simulink model "Sim_Helikopter"  (R2020b)
settings: Solver=ode113  StartTime=0.0  StopTime=50  RelTol=1e-2  EnableMultiTasking=on
PostLoadFcn:
  | , if any(exist('dsrtsu_mdlpostloadfcn', 'file') == [2, 3, 6]), try dsrtsu_mdlpostloadfcn('Execute', bdroot); catch fprintf('Error in PostLoadFcn (dsrtsu_mdlpostloadfcn) for model "%s":\n %s\n', bdroot, lasterr); end, end,
values from neighbouring files (symbols this model uses):
  initCond = [0,0,q20,0,0,0,0,0,0,0,0,0]'    [set_parameter_vollstaendigesModell.m]
undefined symbols (not defined in the file or in its folder): regPar, sysPar, Ta
libraries: simulink x1
settings Model: DSRTSU_INTERNAL_RTI_VER=480  DSRTSU_INTERNAL_RTI_TYPE=rti1202  DSRTSU_INTERNAL_RTIFPGA=70  ExtModeArmWhenConnect=off  Creator=tk  LastModifiedBy=paul
settings DataIOCC: LimitDataPoints=on  SaveFormat=Array  SignalLoggingSaveFormat=ModelDataLogs  ReturnWorkspaceOutputs=off  SignalLoggingName=sigsOut
settings OptimizationCC: ConditionallyExecuteInputs=off  OptimizeBlockIOStorage=off  BufferReuse=off  GlobalBufferReuse=off  ExpressionFolding=off  ExpressionDepthLimit=2147483647  LocalBlockOutputs=off  InitFltsAndDblsToZero=on  LifeSpan=inf  OptimizeDataStoreBuffers=off  BusAssignmentInplaceUpdate=off
settings DebuggingCC: SaveWithParameterizedLinksMsg=none  UnderspecifiedInitializationDetection=Classic  MergeDetectMultiDrivingBlocksExec=none  SignalResolutionControl=TryResolveAllWithWarning  MultiTaskDSMMsg=warning  MultiTaskCondExecSysMsg=none  FcnCallInpInsideContextMsg=warning  AllowSymbolicDim=off  StateNameClashWarn=warning  SFUnexpectedBacktrackingDiag=warning  SFNoUnconditionalDefaultTransitionDiag=warning  SFExecutionAtInitializationDiag=none  ArithmeticOperatorsInVariantConditions=warning
settings HardwareCC: ProdBitPerPointer=32  ProdBitPerSizeT=32  ProdBitPerPtrDiffT=32  ProdLargestAtomicFloat=None  ProdIntDivRoundTo=Undefined  ProdEndianess=Unspecified  ProdWordSize=32  ProdHWDeviceType=32-bit Generic  TargetBitPerLong=64  TargetBitPerPointer=64  TargetBitPerSizeT=64  TargetBitPerPtrDiffT=64  TargetLongLongMode=on  TargetIntDivRoundTo=Zero  TargetEndianess=LittleEndian  TargetWordSize=64  TargetHWDeviceType=MATLAB Host  ProdEqTarget=off
settings ModelReferenceCC: PropagateSignalLabelsOutOfModel=off
settings SFSimCC: SimUseLocalCustomCode=off  SimParseCustomCode=off  CustomCodeUndefinedFunction=UseInterfaceOnly
settings RTWCC: Description=S-function Target  SystemTargetFile=rtwsfcn.tlc  TemplateMakefile=rtwsfcn_default_tmf  RetainRTWFile=on  RTWUseLocalCustomCode=off  RTWCompilerOptimization=on
settings CodeAppCC: StateflowObjectComments=on
settings STFCustomTargetCC: ModelReferenceCompliant=off  CompOptLevelCompliant=on  ConcurrentExecutionCompliant=off  MATLABClassNameForMDSCustomization=Simulink.SoftwareTarget.TargetSpecificTriggerConfigurationBase  CPPClassGenCompliant=off  SystemTargetFile=rtwsfcn.tlc
settings ConfigComp: CovMetricSettings=dw  CovSaveCumulativeToWorkspaceVar=on  CovSaveSingleToWorkspaceVar=on  CovExternalEMLEnable=off

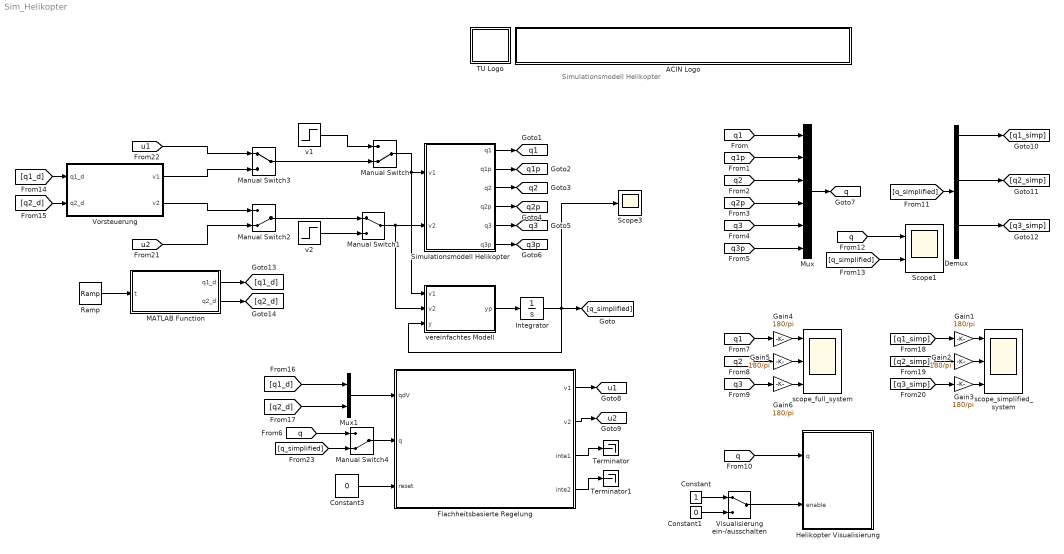
== system Sim_Helikopter ==
  note: Simulationsmodell Helikopter
  ACIN Logo : Subsystem
      mask init:
      | s = get_param(gcb,'UserData');
      mask Display:
      | image(s.logo,[0 0 439 45]);
      | %axis image
  Constant : Constant
  Constant1 : Constant  Value=0
  Constant3 : Constant  Value=0
  Demux : Demux  Outputs=6
  Flachheitsbasierte Regelung : MATLAB Function  TreatAsAtomicUnit=on
  Gain{1..6} (6 alike) : Gain  Gain=180/pi  SaturateOnIntegerOverflow=on  OutDataTypeStr=Inherit: Same as input  ParamDataTypeStr=Inherit: Same as input
  Helikopter Visualisierung : MATLAB Function  TreatAsAtomicUnit=on
  Integrator : Integrator  InitialCondition=sysPar.qR
  MATLAB Function : MATLAB Function  TreatAsAtomicUnit=on
  Manual Switch : ManualSwitch  CurrentSetting=0
  Manual Switch1 : ManualSwitch
  Manual Switch2 : ManualSwitch  CurrentSetting=0
  Manual Switch3 : ManualSwitch
  Manual Switch4 : ManualSwitch  CurrentSetting=0
  Mux : Mux  Inputs=6
  Mux1 : Mux  Inputs=2
  Ramp : simulink/Sources/Ramp  slope=1  start=0  InitialOutput=0
  Scope1 : Scope  NumInputPorts=2
  Scope3 : Scope
  Simulationsmodell Helikopter : Subsystem
      settings: MinAlgLoopOccurrences=on
  TU Logo : Subsystem
      mask init:
      | s = get_param(gcb,'UserData');
      mask Display: image(s.logo,[0 0 45 45]);
  Terminator : Terminator
  Terminator1 : Terminator
  Visualisierung ein-/ausschalten : ManualSwitch
  Vorsteuerung : MATLAB Function  TreatAsAtomicUnit=on
  scope_full_system : Scope  NumInputPorts=3
  scope_simplified_system : Scope  NumInputPorts=3
  v1 : Step  After=.5  SampleTime=0
  v2 : Step  After=0  SampleTime=0
  vereinfachtes Modell : MATLAB Function  TreatAsAtomicUnit=on
  tag scope: q1=global, q1p=global, q2=global, q2p=global, q3=global, q3p=global, q=global, u1=global, u2=global
  wires:
  Gain4/1 -> scope_full_system/1
  Gain5/1 -> scope_full_system/2
  Gain6/1 -> scope_full_system/3
  Flachheitsbasierte Regelung/1(v1) -> [u1]
  Flachheitsbasierte Regelung/2(v2) -> [u2]
  Constant3/1 -> Flachheitsbasierte Regelung/3(reset)
  Simulationsmodell Helikopter/1(q1) -> [q1]
  Simulationsmodell Helikopter/2(q1p) -> [q1p]
  Simulationsmodell Helikopter/3(q2) -> [q2]
  Simulationsmodell Helikopter/4(q2p) -> [q2p]
  Simulationsmodell Helikopter/5(q3) -> [q3]
  Simulationsmodell Helikopter/6(q3p) -> [q3p]
  Mux/1 -> [q]
  [q1] -> Mux/1
  [q1p] -> Mux/2
  [q2] -> Mux/3
  [q2p] -> Mux/4
  [q3] -> Mux/5
  [q3p] -> Mux/6
  [q1] -> Gain4/1
  [q2] -> Gain5/1
  [q3] -> Gain6/1
  Flachheitsbasierte Regelung/3(inte1) -> Terminator/1
  Flachheitsbasierte Regelung/4(inte2) -> Terminator1/1
  Visualisierung ein-/ausschalten/1 -> Helikopter Visualisierung/2(enable)
  Constant/1 -> Visualisierung ein-/ausschalten/1
  [q] -> Helikopter Visualisierung/1(q)
  Constant1/1 -> Visualisierung ein-/ausschalten/2
  vereinfachtes Modell/1(yp) -> Integrator/1
  Integrator/1 -> Scope3/1, [q_simplified], vereinfachtes Modell/3(y)
  [q_simplified] -> Demux/1
  Demux/1 -> [q1_simp]
  Demux/3 -> [q2_simp]
  Demux/5 -> [q3_simp]
  [q] -> Scope1/1
  [q_simplified] -> Scope1/2
  Ramp/1 -> MATLAB Function/1(t)
  MATLAB Function/1(q1_d) -> [q1_d]
  MATLAB Function/2(q2_d) -> [q2_d]
  [q1_d] -> Vorsteuerung/1(q1_d)
  [q2_d] -> Vorsteuerung/2(q2_d)
  Manual Switch/1 -> vereinfachtes Modell/1(v1), Simulationsmodell Helikopter/1(v1)
  v1/1 -> Manual Switch/1
  Manual Switch1/1 -> vereinfachtes Modell/2(v2), Simulationsmodell Helikopter/2(v2)
  v2/1 -> Manual Switch1/2
  Mux1/1 -> Flachheitsbasierte Regelung/1(qdV)
  [q1_d] -> Mux1/1
  [q2_d] -> Mux1/2
  Gain3/1 -> scope_simplified_system/3
  [q3_simp] -> Gain3/1
  Gain2/1 -> scope_simplified_system/2
  Gain1/1 -> scope_simplified_system/1
  [q1_simp] -> Gain1/1
  [q2_simp] -> Gain2/1
  Manual Switch2/1 -> Manual Switch1/1
  Manual Switch3/1 -> Manual Switch/2
  [u1] -> Manual Switch3/1
  Vorsteuerung/1(v1) -> Manual Switch3/2
  [u2] -> Manual Switch2/2
  Vorsteuerung/2(v2) -> Manual Switch2/1
  [q_simplified] -> Manual Switch4/2
  Manual Switch4/1 -> Flachheitsbasierte Regelung/2(q)
  [q] -> Manual Switch4/1

== system Sim_Helikopter/ACIN Logo ==

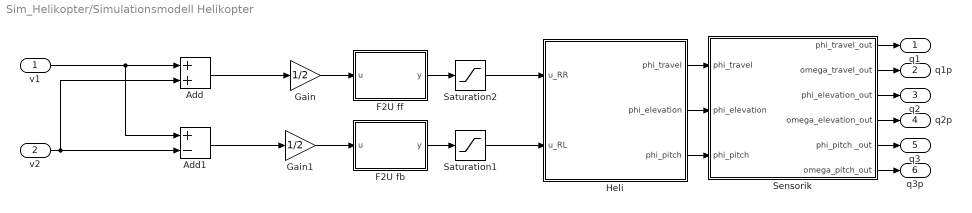
== system Sim_Helikopter/Simulationsmodell Helikopter ==
  v1 : Inport
  v2 : Inport  Port=2
  Add : Sum
  Add1 : Sum  Inputs=+-
  F2U fb : MATLAB Function  TreatAsAtomicUnit=on
  F2U ff : MATLAB Function  TreatAsAtomicUnit=on
  Gain : Gain  Gain=1/2
  Gain1 : Gain  Gain=1/2
  Heli : Subsystem
  Saturation1 : Saturate  UpperLimit=15  LowerLimit=-15
  Saturation2 : Saturate  UpperLimit=15  LowerLimit=-15
  Sensorik : Subsystem
  q1 : Outport  VectorParamsAs1DForOutWhenUnconnected=off
  q1p : Outport  Port=2  VectorParamsAs1DForOutWhenUnconnected=off
  q2 : Outport  Port=3  VectorParamsAs1DForOutWhenUnconnected=off
  q2p : Outport  Port=4  VectorParamsAs1DForOutWhenUnconnected=off
  q3 : Outport  Port=5  VectorParamsAs1DForOutWhenUnconnected=off
  q3p : Outport  Port=6  VectorParamsAs1DForOutWhenUnconnected=off
  wires:
  Saturation1/1 -> Heli/2(u_RL)
  Saturation2/1 -> Heli/1(u_RR)
  Heli/1(phi_travel) -> Sensorik/1(phi_travel)
  Heli/2(phi_elevation) -> Sensorik/2(phi_elevation)
  Heli/3(phi_pitch) -> Sensorik/3(phi_pitch)
  Sensorik/1(phi_travel_out) -> q1/1
  Sensorik/2(omega_travel_out) -> q1p/1
  Sensorik/3(phi_elevation_out) -> q2/1
  Sensorik/4(omega_elevation_out) -> q2p/1
  Sensorik/5(phi_pitch _out) -> q3/1
  Sensorik/6(omega_pitch_out) -> q3p/1
  v1/1 -> Add/1, Add1/1
  v2/1 -> Add/2, Add1/2
  Add/1 -> Gain/1
  Add1/1 -> Gain1/1
  Gain/1 -> F2U ff/1(u)
  Gain1/1 -> F2U fb/1(u)
  F2U ff/1(y) -> Saturation2/1
  F2U fb/1(y) -> Saturation1/1

== system Sim_Helikopter/TU Logo ==

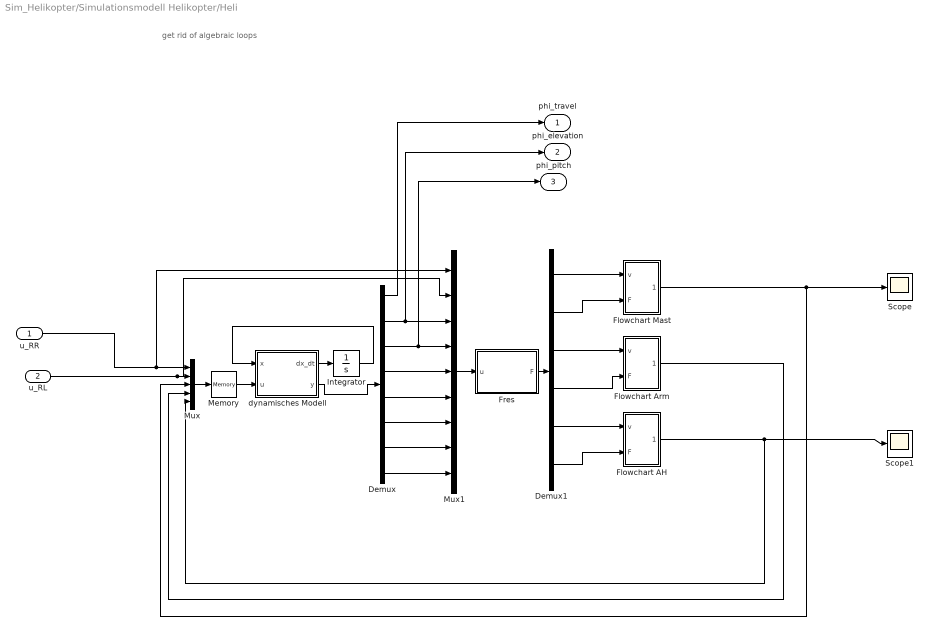
== system Sim_Helikopter/Simulationsmodell Helikopter/Heli ==
  note: get rid of algebraic loops
  u_RR : Inport
  u_RL : Inport  Port=2
  Demux : Demux  Outputs=8
      settings: DisplayOption=none
  Demux1 : Demux  Outputs=6
      settings: DisplayOption=none
  Flowchart AH : Subsystem
  Flowchart Arm : Subsystem
  Flowchart Mast : Subsystem
  Fres : MATLAB Function  TreatAsAtomicUnit=on
  Integrator : Integrator  InitialCondition=initCond
  Memory : Memory
  Mux : Mux  Inputs=5
  Mux1 : Mux  Inputs=9
  Scope : Scope
  Scope1 : Scope
  dynamisches Modell : MATLAB Function  TreatAsAtomicUnit=on
  phi_travel : Outport  VectorParamsAs1DForOutWhenUnconnected=off
  phi_elevation : Outport  Port=2  VectorParamsAs1DForOutWhenUnconnected=off
  phi_pitch : Outport  Port=3  VectorParamsAs1DForOutWhenUnconnected=off
  wires:
  Demux/1 -> phi_travel/1
  u_RR/1 -> Mux1/1, Mux/1
  u_RL/1 -> Mux1/2, Mux/2
  Demux1/6 -> Flowchart AH/2(F)
  Demux1/5 -> Flowchart AH/1(v)
  Demux1/4 -> Flowchart Arm/2(F)
  Demux1/3 -> Flowchart Arm/1(v)
  Demux1/2 -> Flowchart Mast/2(F)
  Demux1/1 -> Flowchart Mast/1(v)
  Fres/1(F) -> Demux1/1
  Mux1/1 -> Fres/1(u)
  Demux/2 -> Mux1/3, phi_elevation/1
  Demux/3 -> Mux1/4, phi_pitch/1
  Demux/4 -> Mux1/5
  Demux/5 -> Mux1/6
  Demux/6 -> Mux1/7
  Demux/7 -> Mux1/8
  Demux/8 -> Mux1/9
  dynamisches Modell/2(y) -> Demux/1
  Mux/1 -> Memory/1
  dynamisches Modell/1(dx_dt) -> Integrator/1
  Integrator/1 -> dynamisches Modell/1(x)
  Flowchart AH/1(Out1) -> Scope1/1, Mux/5
  Flowchart Arm/1(Out1) -> Mux/4
  Flowchart Mast/1(Out1) -> Mux/3, Scope/1
  Memory/1 -> dynamisches Modell/2(u)

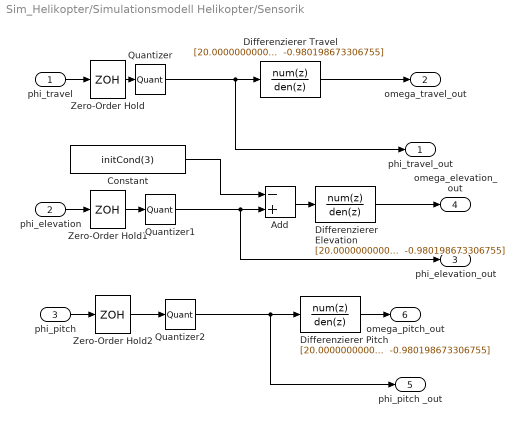
== system Sim_Helikopter/Simulationsmodell Helikopter/Sensorik ==
  phi_travel : Inport
  phi_elevation : Inport  Port=2
  phi_pitch : Inport  Port=3
  Add : Sum  Inputs=-+
  Constant : Constant  Value=initCond(3)
  Differenzierer Elevation : DiscreteTransferFcn  Numerator=[20.000000000000000 -19.999999999999996]  Denominator="[1.000000000000000  -0.980198673306755]"  SampleTime=1e-3
  Differenzierer Pitch : DiscreteTransferFcn  Numerator=[20.000000000000000 -19.999999999999996]  Denominator="[1.000000000000000  -0.980198673306755]"  SampleTime=1e-3
  Differenzierer Travel : DiscreteTransferFcn  Numerator=[20.000000000000000 -19.999999999999996]  Denominator="[1.000000000000000  -0.980198673306755]"  SampleTime=1e-3
  Quantizer : Quantizer  QuantizationInterval=2*pi/2^13
  Quantizer1 : Quantizer  QuantizationInterval=2*pi/4096
  Quantizer2 : Quantizer  QuantizationInterval=2*pi/4096
  Zero-Order Hold : ZeroOrderHold  SampleTime=1e-3
  Zero-Order Hold1 : ZeroOrderHold  SampleTime=1e-3
  Zero-Order Hold2 : ZeroOrderHold  SampleTime=1e-3
  phi_travel_out : Outport  VectorParamsAs1DForOutWhenUnconnected=off
  omega_travel_out : Outport  Port=2  VectorParamsAs1DForOutWhenUnconnected=off
  phi_elevation_out : Outport  Port=3  VectorParamsAs1DForOutWhenUnconnected=off
  omega_elevation_out : Outport  Port=4  VectorParamsAs1DForOutWhenUnconnected=off
  phi_pitch _out : Outport  Port=5  VectorParamsAs1DForOutWhenUnconnected=off
  omega_pitch_out : Outport  Port=6  VectorParamsAs1DForOutWhenUnconnected=off
  wires:
  Add/1 -> Differenzierer Elevation/1
  Constant/1 -> Add/1
  Zero-Order Hold/1 -> Quantizer/1
  Quantizer/1 -> Differenzierer Travel/1, phi_travel_out/1
  Zero-Order Hold1/1 -> Quantizer1/1
  Quantizer1/1 -> Add/2, phi_elevation_out/1
  Zero-Order Hold2/1 -> Quantizer2/1
  Quantizer2/1 -> phi_pitch _out/1, Differenzierer Pitch/1
  Differenzierer Travel/1 -> omega_travel_out/1
  phi_travel/1 -> Zero-Order Hold/1
  Differenzierer Elevation/1 -> omega_elevation_out/1
  phi_elevation/1 -> Zero-Order Hold1/1
  Differenzierer Pitch/1 -> omega_pitch_out/1
  phi_pitch/1 -> Zero-Order Hold2/1

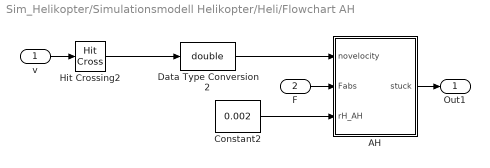
== system Sim_Helikopter/Simulationsmodell Helikopter/Heli/Flowchart AH ==
  v : Inport
  F : Inport  Port=2
  AH : Stateflow chart  TreatAsAtomicUnit=on
  Constant2 : Constant  Value=0.002
  Data Type Conversion2 : DataTypeConversion  OutDataTypeStr=double  SaturateOnIntegerOverflow=on  RndMeth=Zero
  Hit Crossing2 : HitCross  ZeroCross=off
  Out1 : Outport  VectorParamsAs1DForOutWhenUnconnected=off
  wires:
  AH/1(stuck) -> Out1/1
  F/1 -> AH/2(Fabs)
  v/1 -> Hit Crossing2/1
  Constant2/1 -> AH/3(rH_AH)
  Data Type Conversion2/1 -> AH/1(novelocity)
  Hit Crossing2/1 -> Data Type Conversion2/1

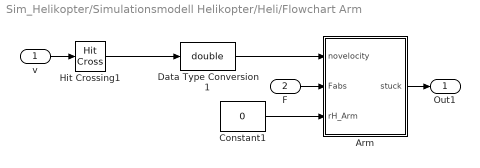
== system Sim_Helikopter/Simulationsmodell Helikopter/Heli/Flowchart Arm ==
  v : Inport
  F : Inport  Port=2
  Arm : Stateflow chart  TreatAsAtomicUnit=on
  Constant1 : Constant  Value=0
  Data Type Conversion1 : DataTypeConversion  OutDataTypeStr=double  SaturateOnIntegerOverflow=on  RndMeth=Zero
  Hit Crossing1 : HitCross  ZeroCross=off
  Out1 : Outport  VectorParamsAs1DForOutWhenUnconnected=off
  wires:
  Arm/1(stuck) -> Out1/1
  F/1 -> Arm/2(Fabs)
  v/1 -> Hit Crossing1/1
  Hit Crossing1/1 -> Data Type Conversion1/1
  Data Type Conversion1/1 -> Arm/1(novelocity)
  Constant1/1 -> Arm/3(rH_Arm)

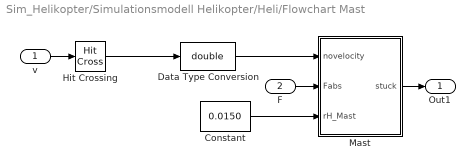
== system Sim_Helikopter/Simulationsmodell Helikopter/Heli/Flowchart Mast ==
  v : Inport
  F : Inport  Port=2
  Constant : Constant  Value=0.0150
  Data Type Conversion : DataTypeConversion  OutDataTypeStr=double  SaturateOnIntegerOverflow=on  RndMeth=Zero
  Hit Crossing : HitCross  ZeroCross=off
  Mast : Stateflow chart  TreatAsAtomicUnit=on
  Out1 : Outport  VectorParamsAs1DForOutWhenUnconnected=off
  wires:
  Mast/1(stuck) -> Out1/1
  F/1 -> Mast/2(Fabs)
  v/1 -> Hit Crossing/1
  Constant/1 -> Mast/3(rH_Mast)
  Data Type Conversion/1 -> Mast/1(novelocity)
  Hit Crossing/1 -> Data Type Conversion/1

== matlab function Sim_Helikopter/Simulationsmodell Helikopter/Heli/dynamisches Modell ==
  data: x input; u input; dx_dt output; p parameter; y output
function [dx_dt, y]= fcn(x, u, p)
%#codegen

[dx_dt, y] = heli_haft_mfun(x,u,p);

== matlab function Sim_Helikopter/Helikopter Visualisierung ==
  settings: updateMethod=DISCRETE  sampleTime=0.1
  data: q input; enable input
function visualization(q, enable)
  %Die Framerate wird durch die Sampling Time des Blocks vorgegeben.

  persistent ini; if isempty(ini);    ini = 0;    end
  persistent z12; if isempty(z12);    z12 = 1;    end
  persistent x23; if isempty(x23);    x23 = 1;    end
  persistent xh;  if isempty(xh);     xh = 1;     end
  persistent yh;  if isempty(yh);     yh = 1;     end
  persistent zh;  if isempty(zh);     zh = 1;     end
  persistent ph;  if isempty(ph);     ph = 1;     end
  
  if ~ini
    if(enable)
      h=figure(100);
      clf('reset');
      plot3(-2, -2, 0);
      plot3( 2,  2, 0);
      plot3(-2,  2, 0);
      plot3( 2, -2, 0);
      axis([-2 2 -2 2 0 1]);
      xlabel('x');
      ylabel('y');
      zlabel('-z');

      r  = 0.1;
      yn = 0.2:0.01:0.4;
      yp = 0.4:-0.01:0.2;
      a  = abs(r^2 - (yn - 0.3).^2);
      xn = -sqrt(a);
      xp =  sqrt(a);

      y2 = [yn'; yp'];
      x2 = [xn'; xp'];
      z2 = zeros(size(x2));

      yn = -0.2:-0.01:-0.4;
      yp = -0.4:0.01:-0.2;
      b  = abs(r^2 - (yn + 0.3).^2);
      xn = -sqrt(b);
      xp =  sqrt(b);

      y1 = [yn'; yp'];
      x1 = [xn'; xp'];
      z1 = zeros(size(x1));

      xh = [x1', x2'];
      yh = [y1', y2'];
      zh = [z1', z2'];
      ph = [xh; yh; zh; ones(size(zh))];
    else
      h=findobj('type','figure','Number',100);
      if(~isempty(h))
        close(h);
      end
    end
    ini = 1;
  end
  
  if(enable)
    q1=q(1);
    q2=q(3);
    q3=q(5);
    
    T02 = [-sin(q1) * cos(q2) -cos(q1) -sin(q1) * sin(q2) 0; cos(q1) * cos(q2) -sin(q1) cos(q1) * sin(q2) 0; -sin(q2) 0 cos(q2) z12; 0 0 0 1;];
    T03 = [-sin(q1) * cos(q2) cos(q1) * cos(q3) + sin(q1) * sin(q2) * sin(q3) -cos(q1) * sin(q3) + sin(q1) * sin(q2) * cos(q3) -sin(q1) * cos(q2) * x23; cos(q1) * cos(q2) sin(q1) * cos(q3) - cos(q1) * sin(q2) * sin(q3) -sin(q1) * sin(q3) - cos(q1) * sin(q2) * cos(q3) cos(q1) * cos(q2) * x23; -sin(q2) -cos(q2) * sin(q3) -cos(q2) * cos(q3) -sin(q2) * x23 + z12; 0 0 0 1;];

    clf('reset');
    % Nullzeiger
    xn = [0;1];
    yn = [0;0];
    zn = [0;0];
    plot3(xn, yn, zn);
    hold on;
    grid on;

    % Staender
    p0 = [0; 0; 0];
    p1 = [0; 0; 1];    
    lines = [p0';p1'];
    xs = lines(1:2,1);
    ys = lines(1:2,2);
    zs = lines(1:2,3);
    plot3(xs, ys, zs);

    % Balken
    p0 = T02*[1; 0; 0; 1];
    p1 = T02*[-1; 0; 0; 1];    
    lines = [p0(1:3)';p1(1:3)'];
    xb = lines(1:2,1);
    yb = lines(1:2,2);
    zb = lines(1:2,3);
    plot3(xb, yb, zb);

    % Helicopter
    lines = T03*ph;% [0; 0.2; 0; 1];
    % p1 = T03*[0; -0.2; 0; 1];    
    % lines = [p0(1:3)';p1(1:3)'];
    xh = lines(1,:);
    yh = lines(2,:);
    zh = lines(3,:);
    plot3(xh, yh, zh);

    plot3(-2, -2, 0);
    plot3( 2,  2, 0);
    plot3(-2,  2, 0);
    plot3( 2, -2, 0);
    axis([-2 2 -2 2 0 2]);

    drawnow
  end
end

== matlab function Sim_Helikopter/MATLAB Function ==
  data: t input; q1_d output; q2_d output; sysPar parameter
function [q1_d,q2_d] = Trajektorie(t,sysPar)
    
   
    beta5 = 126; beta6 = -420; beta7 = 540; beta8 = -315; beta9 = 70;
    
    % Startpunkt -> Ruhelage
    q1_0 = sysPar.qR(1);
    q2_0 = sysPar.qR(3);
    
    % Zeitpunkte und Endpunkte laut Angabe
    T1 = 5;
    T2 = 10;
    
    q1_end = 2*pi;
    q2_end = 0;

    
    q1_d = [q1_0; zeros(4,1)];
    q2_d = [q2_0; zeros(4,1)];
    
    % Ruhelage
    if (t > 0) && (t <= T1)
        q2_d(1) = q2_0 + (q2_end - q2_0) * (beta5 * t ^ 5 / T1 ^ 5 + beta6 * t ^ 6 / T1 ^ 6 + beta7 * t ^ 7 / T1 ^ 7 + beta8 * t ^ 8 / T1 ^ 8 + beta9 * t ^ 9 / T1 ^ 9);
        q2_d(5) = (q2_end - q2_0) * (120 * beta5 * t / T1 ^ 5 + 360 * beta6 * t ^ 2 / T1 ^ 6 + 840 * beta7 * t ^ 3 / T1 ^ 7 + 1680 * beta8 * t ^ 4 / T1 ^ 8 + 3024 * beta9 * t ^ 5 / T1 ^ 9);
        q2_d(4) = (q2_end - q2_0) * (60 * beta5 * t ^ 2 / T1 ^ 5 + 120 * beta6 * t ^ 3 / T1 ^ 6 + 210 * beta7 * t ^ 4 / T1 ^ 7 + 336 * beta8 * t ^ 5 / T1 ^ 8 + 504 * beta9 * t ^ 6 / T1 ^ 9);
        q2_d(3) = (q2_end - q2_0) * (20 * beta5 * t ^ 3 / T1 ^ 5 + 30 * beta6 * t ^ 4 / T1 ^ 6 + 42 * beta7 * t ^ 5 / T1 ^ 7 + 56 * beta8 * t ^ 6 / T1 ^ 8 + 72 * beta9 * t ^ 7 / T1 ^ 9);
        q2_d(2) = (q2_end - q2_0) * (5 * beta5 * t ^ 4 / T1 ^ 5 + 6 * beta6 * t ^ 5 / T1 ^ 6 + 7 * beta7 * t ^ 6 / T1 ^ 7 + 8 * beta8 * t ^ 7 / T1 ^ 8 + 9 * beta9 * t ^ 8 / T1 ^ 9);
    elseif t > T1
        q2_d = [q2_end; zeros(4,1)];
    else
        q2_d = [q2_0; zeros(4,1)];
    end
        
    if (t > T1) && (t <= T1 + T2)
        q1_d(1) = q1_0 + (q1_end - q1_0) * (beta5 * (t - T1) ^ 5 / T2 ^ 5 + beta6 * (t - T1) ^ 6 / T2 ^ 6 + beta7 * (t - T1) ^ 7 / T2 ^ 7 + beta8 * (t - T1) ^ 8 / T2 ^ 8 + beta9 * (t - T1) ^ 9 / T2 ^ 9);
        q1_d(5) = (q1_end - q1_0) * (120 * beta5 * (t - T1) / T2 ^ 5 + 360 * beta6 * (t - T1) ^ 2 / T2 ^ 6 + 840 * beta7 * (t - T1) ^ 3 / T2 ^ 7 + 1680 * beta8 * (t - T1) ^ 4 / T2 ^ 8 + 3024 * beta9 * (t - T1) ^ 5 / T2 ^ 9);
        q1_d(4) = (q1_end - q1_0) * (60 * beta5 * (t - T1) ^ 2 / T2 ^ 5 + 120 * beta6 * (t - T1) ^ 3 / T2 ^ 6 + 210 * beta7 * (t - T1) ^ 4 / T2 ^ 7 + 336 * beta8 * (t - T1) ^ 5 / T2 ^ 8 + 504 * beta9 * (t - T1) ^ 6 / T2 ^ 9);
        q1_d(3) = (q1_end - q1_0) * (20 * beta5 * (t - T1) ^ 3 / T2 ^ 5 + 30 * beta6 * (t - T1) ^ 4 / T2 ^ 6 + 42 * beta7 * (t - T1) ^ 5 / T2 ^ 7 + 56 * beta8 * (t - T1) ^ 6 / T2 ^ 8 + 72 * beta9 * (t - T1) ^ 7 / T2 ^ 9);
        q1_d(2) = (q1_end - q1_0) * (5 * beta5 * (t - T1) ^ 4 / T2 ^ 5 + 6 * beta6 * (t - T1) ^ 5 / T2 ^ 6 + 7 * beta7 * (t - T1) ^ 6 / T2 ^ 7 + 8 * beta8 * (t - T1) ^ 7 / T2 ^ 8 + 9 * beta9 * (t - T1) ^ 8 / T2 ^ 9);
    elseif t > (T1 + T2)
        q1_d = [q1_end; zeros(4,1)];
    else
        q1_d = [q1_0; zeros(4,1)];
    end
end

== matlab function Sim_Helikopter/Simulationsmodell Helikopter/F2U ff ==
  data: u input; y output
function y = fcn(u)
%#codegen

y = F2U(u(1));

== stateflow chart Sim_Helikopter/Simulationsmodell Helikopter/Heli/Flowchart AH/AH ==
  state stuck/
    entry: stuck=1;
  state sliding/
    entry: stuck=0;
  (default) -> stuck
  sliding -> stuck : [novelocity & fabs(Fabs)<rH_AH]
  stuck -> sliding : [fabs(Fabs)>rH_AH]
  data: novelocity input boolean; Fabs input double; stuck output double; rH_AH input double

== stateflow chart Sim_Helikopter/Simulationsmodell Helikopter/Heli/Flowchart Arm/Arm ==
  state stuck/
    entry: stuck=1;
  state sliding/
    entry: stuck=0;
  (default) -> stuck
  sliding -> stuck : [novelocity & fabs(Fabs)<rH_Arm]
  stuck -> sliding : [fabs(Fabs)>rH_Arm]
  data: novelocity input boolean; Fabs input double; stuck output double; rH_Arm input double

== matlab function Sim_Helikopter/Flachheitsbasierte Regelung ==
  settings: updateMethod=DISCRETE  sampleTime=Ta
  data: qdV input; q input; sysPar parameter; regPar parameter; reset input; v1 output; v2 output; Ta parameter; inte1 output; inte2 output
function [v1,v2,inte1,inte2] = FLATreg(qdV,q,sysPar,regPar,reset,Ta)
%
% Ta ....... Abtastzeit
% sysPar ... Systemparameter
% regPar ... Reglerparameter
% q ........ Messgrößen
% qdV ...... Sollgrößen aus Trajektorienvorgabe für q1 und q2
% reset .... Reset für dSpace
%
% Persistent Variablen für Integration des Fehlers 
persistent e1I
if isempty(e1I) e1I = double(0); end
persistent e2I
if isempty(e2I) e2I = double(0); end

% Reset der Integratoren für die Fehler
if reset
    e1I=0.0;
    e2I=0.0;
end

% Messgrößen 
q1 = q(1);
q1p= q(2);
q2 = q(3);
q2p= q(4);
q3 = q(5);
q3p= q(6);

% Systemparameter
a1 = sysPar.a1;
a2 = sysPar.a2;
a3 = sysPar.a3;
b1 = sysPar.b1;
b2 = sysPar.b2;
b3 = sysPar.b3;

% Auslesen der Reglerparameter
k13 = regPar.k13;
k12 = regPar.k12;
k11 = regPar.k11;
k10 = regPar.k10;
k1I = regPar.k1I;
k21 = regPar.k21;
k20 = regPar.k20;
k2I = regPar.k2I;

% Sollgrößen mit zeitlichen Ableitungen
q1d     = qdV(1);
q1pd    = qdV(2);
q1ppd   = qdV(3);
q1pppd  = qdV(4);
q1ppppd = qdV(5);

q2d     = qdV(6);
q2pd    = qdV(7);
q2ppd   = qdV(8);
q2pppd  = qdV(9);
q2ppppd = qdV(10);


% Integration der Fehler: Hier bitte Integrator (Euler-Vorwärts) für Fehler einfügen!
e1 = q1 - q1d;
e2 = q2 - q2d;

% Euler-vorwärtsverfahren
e1I = e1I + Ta*e1;
e2I = e2I + Ta*e2;

% Quasi-statische Zustandsrückführung Parameter anpassung
w1 = q1ppppd;
w2 = q2ppd;
w2p = q2pppd;
w2pp = q2ppppd;
omega2 = q2p;
omega3 = q3p;

% Fehlerdynamik
q1pp = b1 * cos(q2) * sin(q3) * w2 / b2 / cos(q3) - b1 * cos(q2) * sin(q3) * (a1 * sin(q2) + a2 * cos(q2)) / b2 / cos(q3);
q1ppp = -b1 * sin(q2) * sin(q3) / b2 / cos(q3) * omega2 * w2 + (b1 * cos(q2) / b2 + b1 * cos(q2) * sin(q3) ^ 2 / b2 / cos(q3) ^ 2) * omega3 * w2 + (b1 * sin(q2) * sin(q3) * (a1 * sin(q2) + a2 * cos(q2)) / b2 / cos(q3) - b1 * cos(q2) * sin(q3) * (a1 * cos(q2) - a2 * sin(q2)) / b2 / cos(q3)) * omega2 + (-b1 * cos(q2) * (a1 * sin(q2) + a2 * cos(q2)) / b2 - b1 * cos(q2) * sin(q3) ^ 2 * (a1 * sin(q2) + a2 * cos(q2)) / b2 / cos(q3) ^ 2) * omega3 + b1 * cos(q2) * sin(q3) / b2 / cos(q3) * w2p;

e1p = q1p - q1pd;
e1pp = q1pp - q1ppd;
e1ppp = q1ppp - q1pppd;

e2p = q2p - q2pd;



% Lösung der Quasizustandsrückführung
if 0
v1 = -(a1 * sin(q2) + a2 * cos(q2) - w2) / b2 / cos(q3);
v2 = -(w1 * b2 * cos(q3) ^ 3 + sin(q3) * sin(q2) * cos(q3) ^ 2 * b1 * w2 ^ 2 + 0.2e1 * sin(q3) * cos(q2) ^ 2 * a2 * b1 * omega3 ^ 2 + 0.2e1 * sin(q3) * cos(q3) ^ 2 * a2 * b1 * omega2 ^ 2 - sin(q3) * cos(q2) * cos(q3) ^ 2 * b1 * w2pp - 0.2e1 * sin(q3) * cos(q2) * b1 * omega3 ^ 2 * w2 - sin(q3) * cos(q3) ^ 2 * a1 * b1 * w2 - 0.2e1 * cos(q2) * cos(q3) * b1 * omega3 * w2p - 0.2e1 * cos(q3) * a1 * b1 * omega2 * omega3 - 0.4e1 * sin(q3) * cos(q2) ^ 2 * cos(q3) ^ 2 * a2 * b1 * omega2 ^ 2 + sin(q3) * cos(q2) ^ 3 * cos(q3) * a2 * a3 * b1 + 0.2e1 * sin(q3) * cos(q2) ^ 2 * cos(q3) ^ 2 * a1 * b1 * w2 + sin(q3) * cos(q2) * cos(q3) ^ 2 * b1 * omega2 ^ 2 * w2 + 0.2e1 * sin(q3) * sin(q2) * cos(q2) * a1 * b1 * omega3 ^ 2 + 0.2e1 * sin(q3) * sin(q2) * cos(q3) ^ 2 * b1 * omega2 * w2p - sin(q3) * cos(q2) ^ 2 * cos(q3) * a3 * b1 * w2 + 0.4e1 * cos(q2) ^ 2 * cos(q3) * a1 * b1 * omega2 * omega3 + 0.2e1 * sin(q2) * cos(q3) * b1 * omega2 * omega3 * w2 - 0.4e1 * sin(q3) * sin(q2) * cos(q2) * cos(q3) ^ 2 * a1 * b1 * omega2 ^ 2 + sin(q3) * sin(q2) * cos(q2) ^ 2 * cos(q3) * a1 * a3 * b1 - 0.2e1 * sin(q3) * sin(q2) * cos(q2) * cos(q3) ^ 2 * a2 * b1 * w2 - 0.4e1 * sin(q2) * cos(q2) * cos(q3) * a2 * b1 * omega2 * omega3) / b1 / b3 / cos(q3) / cos(q2) / (a1 * sin(q2) + a2 * cos(q2) - w2);


else
% Hier bitte Regelgesetz einfügen!
v1 = -(a2 * cos(q2) + a1 * sin(q2) + k20 * e2 + k2I * e2I + k21 * e2p - w2) / cos(q3) / b2;
v2 = (k10 * e1 * b2 * cos(q3) ^ 3 + k1I * e1I * b2 * cos(q3) ^ 3 + k11 * e1p * b2 * cos(q3) ^ 3 + k12 * e1pp * b2 * cos(q3) ^ 3 + k13 * e1ppp * b2 * cos(q3) ^ 3 - w1 * b2 * cos(q3) ^ 3 - sin(q3) * sin(q2) * cos(q3) ^ 2 * b1 * w2 ^ 2 - 0.2e1 * sin(q3) * cos(q2) ^ 2 * a2 * b1 * omega3 ^ 2 - 0.2e1 * sin(q3) * cos(q3) ^ 2 * a2 * b1 * omega2 ^ 2 + sin(q3) * cos(q2) * cos(q3) ^ 2 * b1 * w2pp + 0.2e1 * sin(q3) * cos(q2) * b1 * omega3 ^ 2 * w2 + sin(q3) * cos(q3) ^ 2 * a1 * b1 * w2 + 0.2e1 * cos(q2) * cos(q3) * b1 * omega3 * w2p + 0.2e1 * cos(q3) * a1 * b1 * omega2 * omega3 + 0.4e1 * sin(q3) * cos(q2) ^ 2 * cos(q3) ^ 2 * a2 * b1 * omega2 ^ 2 - sin(q3) * cos(q2) ^ 3 * cos(q3) * a2 * a3 * b1 - 0.2e1 * sin(q3) * cos(q2) ^ 2 * cos(q3) ^ 2 * a1 * b1 * w2 - sin(q3) * cos(q2) * cos(q3) ^ 2 * b1 * omega2 ^ 2 * w2 - 0.2e1 * sin(q3) * sin(q2) * cos(q2) * a1 * b1 * omega3 ^ 2 - 0.2e1 * sin(q3) * sin(q2) * cos(q3) ^ 2 * b1 * omega2 * w2p + sin(q3) * cos(q2) ^ 2 * cos(q3) * a3 * b1 * w2 - 0.4e1 * cos(q2) ^ 2 * cos(q3) * a1 * b1 * omega2 * omega3 - 0.2e1 * sin(q2) * cos(q3) * b1 * omega2 * omega3 * w2 + 0.4e1 * sin(q3) * sin(q2) * cos(q2) * cos(q3) ^ 2 * a1 * b1 * omega2 ^ 2 - sin(q3) * sin(q2) * cos(q2) ^ 2 * cos(q3) * a1 * a3 * b1 + 0.2e1 * sin(q3) * sin(q2) * cos(q2) * cos(q3) ^ 2 * a2 * b1 * w2 + 0.4e1 * sin(q2) * cos(q2) * cos(q3) * a2 * b1 * omega2 * omega3) / cos(q3) / cos(q2) / b1 / b3 / (a1 * sin(q2) + a2 * cos(q2) - w2);
end


% Ausgabe der Werte der Fehlerintegratoren
inte1 = e1I;
inte2 = e2I;

end

== stateflow chart Sim_Helikopter/Simulationsmodell Helikopter/Heli/Flowchart Mast/Mast ==
  state stuck/
    entry: stuck=1;
  state sliding/
    entry: stuck=0;
  sliding -> stuck : [novelocity & fabs(Fabs)<rH_Mast]
  stuck -> sliding : [fabs(Fabs)>rH_Mast]
  (default) -> sliding
  data: novelocity input boolean; Fabs input double; stuck output double; rH_Mast input double

== matlab function Sim_Helikopter/vereinfachtes Modell ==
  data: v1 input; yp output; v2 input; y input; sysPar parameter
function yp = fcn(v1,v2,y,sysPar)
    
    % import der Parameter
    a1 = sysPar.a1;
    a2 = sysPar.a2;
    a3 = sysPar.a3;
    b1 = sysPar.b1;
    b2 = sysPar.b2;
    b3 = sysPar.b3;
    
    % neue Werte berechnen
    % q1 = y(1);
    q2 = y(3);
    q3 = y(5);
    
    q1p = y(2);
    
    q1pp = b1 * cos(q2) * sin(q3) * v1;
   
    q2p = y(4);
    q2pp = a1 * sin(q2) + a2 * cos(q2) + b2 * cos(q3) * v1;
    
    q3p = y(6);
    q3pp = a3 * cos(q2) * sin(q3) + b3 * v2;
    
    % Ausgangsvektor erstellen
    yp = [q1p q1pp q2p q2pp q3p q3pp];
end

== matlab function Sim_Helikopter/Vorsteuerung ==
  data: q1_d input; v1 output; q2_d input; v2 output; sysPar parameter
function [v1,v2] = Vorsteuerung(q1_d,q2_d,sysPar)
    
    % Parameter einlesen
    a1 = sysPar.a1;
    a2 = sysPar.a2;
    a3 = sysPar.a3;
    
    b1 = sysPar.b1;
    b2 = sysPar.b2;
    b3 = sysPar.b3;
    
    q1 = q1_d(1);
    q1_p = q1_d(2);
    q1_pp = q1_d(3);
    q1_ppp = q1_d(4);
    q1_pppp = q1_d(5);
    
    q2 = q2_d(1);
    q2_p = q2_d(2);
    q2_pp = q2_d(3);
    q2_ppp = q2_d(4);
    q2_pppp = q2_d(5);
    
    % Maple import
    v1 = -0.1e1 / b2 * (a1 * sin(q2) + a2 * cos(q2) - q2_pp) * sqrt(b2 ^ 2 * q1_pp ^ 2 / b1 ^ 2 / cos(q2) ^ 2 / (a1 * sin(q2) + a2 * cos(q2) - q2_pp) ^ 2 + 0.1e1);
    v2 = (0.3e1 * (cos(q2) ^ 2 * q2_pp ^ 3 * b1 ^ 2 / 0.3e1 - cos(q2) ^ 2 * b1 ^ 2 * (a1 * sin(q2) + a2 * cos(q2)) * q2_pp ^ 2 + (b2 ^ 2 * q1_pp ^ 2 / 0.3e1 - ((a1 ^ 2 - a2 ^ 2) * cos(q2) ^ 2 - 0.2e1 * sin(q2) * a1 * a2 * cos(q2) - a1 ^ 2) * b1 ^ 2 * cos(q2) ^ 2) * q2_pp - b2 ^ 2 * (a1 * sin(q2) + a2 * cos(q2)) * q1_pp ^ 2 / 0.3e1 + b1 ^ 2 * cos(q2) ^ 2 * ((a1 ^ 2 * a2 - a2 ^ 3 / 0.3e1) * cos(q2) ^ 3 + sin(q2) * a1 * (a1 ^ 2 - 0.3e1 * a2 ^ 2) * cos(q2) ^ 2 / 0.3e1 - cos(q2) * a1 ^ 2 * a2 - sin(q2) * a1 ^ 3 / 0.3e1)) * b1 * cos(q2) * b2 * q1_pppp + b1 * cos(q2) * b2 * (-q2_pp ^ 2 * cos(q2) ^ 2 * b1 ^ 2 + 0.2e1 * cos(q2) ^ 2 * b1 ^ 2 * (a1 * sin(q2) + a2 * cos(q2)) * q2_pp - b2 ^ 2 * q1_pp ^ 2 + ((a1 ^ 2 - a2 ^ 2) * cos(q2) ^ 2 - 0.2e1 * sin(q2) * a1 * a2 * cos(q2) - a1 ^ 2) * b1 ^ 2 * cos(q2) ^ 2) * q1_pp * q2_pppp + 0.2e1 * cos(q2) * q1_pp * b1 * b2 ^ 3 * (a1 * sin(q2) + a2 * cos(q2) - q2_pp) * q1_ppp ^ 2 - 0.4e1 * (-(-q2_pp ^ 2 * cos(q2) ^ 2 * b1 ^ 2 + 0.2e1 * cos(q2) ^ 2 * b1 ^ 2 * (a1 * sin(q2) + a2 * cos(q2)) * q2_pp + b2 ^ 2 * q1_pp ^ 2 + ((a1 ^ 2 - a2 ^ 2) * cos(q2) ^ 2 - 0.2e1 * sin(q2) * a1 * a2 * cos(q2) - a1 ^ 2) * b1 ^ 2 * cos(q2) ^ 2) * cos(q2) * q2_ppp / 0.2e1 + (-cos(q2) ^ 2 * sin(q2) * q2_pp ^ 3 * b1 ^ 2 / 0.2e1 - 0.2e1 * b1 ^ 2 * cos(q2) ^ 2 * (cos(q2) ^ 2 * a1 - cos(q2) * sin(q2) * a2 - 0.3e1 / 0.4e1 * a1) * q2_pp ^ 2 + (sin(q2) * q1_pp ^ 2 * b2 ^ 2 / 0.2e1 + 0.5e1 * (cos(q2) ^ 3 * a1 * a2 + sin(q2) * (a1 ^ 2 / 0.2e1 - a2 ^ 2 / 0.2e1) * cos(q2) ^ 2 - 0.4e1 / 0.5e1 * cos(q2) * a1 * a2 - 0.3e1 / 0.10e2 * sin(q2) * a1 ^ 2) * b1 ^ 2 * cos(q2) ^ 2) * q2_pp + b2 ^ 2 * (-a1 / 0.2e1 + cos(q2) ^ 2 * a1 - cos(q2) * sin(q2) * a2) * q1_pp ^ 2 + ((a1 ^ 3 - 0.3e1 * a1 * a2 ^ 2) * cos(q2) ^ 4 + (-0.3e1 * a1 ^ 2 * a2 + a2 ^ 3) * sin(q2) * cos(q2) ^ 3 + (-0.3e1 / 0.2e1 * a1 ^ 3 + 0.5e1 / 0.2e1 * a1 * a2 ^ 2) * cos(q2) ^ 2 + 0.2e1 * cos(q2) * sin(q2) * a1 ^ 2 * a2 + a1 ^ 3 / 0.2e1) * b1 ^ 2 * cos(q2) ^ 2) * q2_p) * b1 * b2 * q1_ppp - 0.2e1 * cos(q2) ^ 3 * q1_pp * b1 ^ 3 * b2 * (a1 * sin(q2) + a2 * cos(q2) - q2_pp) * q2_ppp ^ 2 + 0.12e2 * (-cos(q2) ^ 2 * sin(q2) * q2_pp ^ 2 * b1 ^ 2 / 0.6e1 - 0.2e1 / 0.3e1 * b1 ^ 2 * cos(q2) ^ 2 * (-a1 / 0.2e1 + cos(q2) ^ 2 * a1 - cos(q2) * sin(q2) * a2) * q2_pp + sin(q2) * q1_pp ^ 2 * b2 ^ 2 / 0.6e1 + (cos(q2) ^ 3 * a1 * a2 + sin(q2) * (a1 ^ 2 / 0.2e1 - a2 ^ 2 / 0.2e1) * cos(q2) ^ 2 - 0.2e1 / 0.3e1 * cos(q2) * a1 * a2 - sin(q2) * a1 ^ 2 / 0.6e1) * b1 ^ 2 * cos(q2) ^ 2) * b1 * b2 * q2_p * q1_pp * q2_ppp + (cos(q2) ^ 4 * b2 * q1_pp * b1 ^ 3 / (a1 * sin(q2) + a2 * cos(q2) - q2_pp) * (0.1e1 + b2 ^ 2 * q1_pp ^ 2 / b1 ^ 2 / cos(q2) ^ 2 / (a1 * sin(q2) + a2 * cos(q2) - q2_pp) ^ 2) ^ (-0.1e1 / 0.2e1) * a3 + cos(q2) ^ 2 * sin(q2) * b1 ^ 3 * b2 * q1_pp) * q2_pp ^ 4 + 0.4e1 * b1 ^ 3 * cos(q2) * (((-cos(q2) ^ 2 / 0.4e1 + 0.1e1 / 0.2e1) * q2_p ^ 2 + cos(q2) * (cos(q2) ^ 2 * a1 - cos(q2) * sin(q2) * a2 - 0.3e1 / 0.4e1 * a1)) * b2 * q1_pp - cos(q2) ^ 3 * b2 * q1_pp / (a1 * sin(q2) + a2 * cos(q2) - q2_pp) * (0.1e1 + b2 ^ 2 * q1_pp ^ 2 / b1 ^ 2 / cos(q2) ^ 2 / (a1 * sin(q2) + a2 * cos(q2) - q2_pp) ^ 2) ^ (-0.1e1 / 0.2e1) * a3 * (a1 * sin(q2) + a2 * cos(q2))) * q2_pp ^ 3 + 0.6e1 * b1 * (sin(q2) * q1_pp ^ 3 * b2 ^ 3 / 0.6e1 + cos(q2) ^ 2 * b2 ^ 3 * q1_pp ^ 3 / (a1 * sin(q2) + a2 * cos(q2) - q2_pp) * (0.1e1 + b2 ^ 2 * q1_pp ^ 2 / b1 ^ 2 / cos(q2) ^ 2 / (a1 * sin(q2) + a2 * cos(q2) - q2_pp) ^ 2) ^ (-0.1e1 / 0.2e1) * a3 / 0.3e1 - 0.5e1 / 0.3e1 * b1 ^ 2 * cos(q2) * ((-0.2e1 / 0.5e1 * cos(q2) ^ 3 * a2 - 0.2e1 / 0.5e1 * cos(q2) ^ 2 * sin(q2) * a1 + 0.4e1 / 0.5e1 * a2 * cos(q2) + 0.3e1 / 0.5e1 * a1 * sin(q2)) * q2_p ^ 2 + (cos(q2) ^ 3 * a1 * a2 + sin(q2) * (a1 ^ 2 / 0.2e1 - a2 ^ 2 / 0.2e1) * cos(q2) ^ 2 - 0.4e1 / 0.5e1 * cos(q2) * a1 * a2 - 0.3e1 / 0.10e2 * sin(q2) * a1 ^ 2) * cos(q2)) * b2 * q1_pp - cos(q2) ^ 4 * ((a1 ^ 2 - a2 ^ 2) * cos(q2) ^ 2 - 0.2e1 * sin(q2) * a1 * a2 * cos(q2) - a1 ^ 2) * b1 ^ 2 * b2 * q1_pp / (a1 * sin(q2) + a2 * cos(q2) - q2_pp) * (0.1e1 + b2 ^ 2 * q1_pp ^ 2 / b1 ^ 2 / cos(q2) ^ 2 / (a1 * sin(q2) + a2 * cos(q2) - q2_pp) ^ 2) ^ (-0.1e1 / 0.2e1) * a3) * q2_pp ^ 2 - 0.12e2 * b1 * (-(cos(q2) ^ 2 * a1 - cos(q2) * sin(q2) * a2 + cos(q2) * q2_p ^ 2 / 0.2e1 - a1 / 0.2e1) * b2 ^ 3 * q1_pp ^ 3 / 0.6e1 + cos(q2) ^ 2 * b2 ^ 3 * q1_pp ^ 3 / (a1 * sin(q2) + a2 * cos(q2) - q2_pp) * (0.1e1 + b2 ^ 2 * q1_pp ^ 2 / b1 ^ 2 / cos(q2) ^ 2 / (a1 * sin(q2) + a2 * cos(q2) - q2_pp) ^ 2) ^ (-0.1e1 / 0.2e1) * a3 * (a1 * sin(q2) + a2 * cos(q2)) / 0.3e1 + b1 ^ 2 * (((-0.7e1 / 0.2e1 * a1 ^ 2 + 0.7e1 / 0.2e1 * a2 ^ 2) * cos(q2) ^ 4 + 0.7e1 * cos(q2) ^ 3 * sin(q2) * a1 * a2 + (0.11e2 / 0.2e1 * a1 ^ 2 - 0.6e1 * a2 ^ 2) * cos(q2) ^ 2 - 0.8e1 * sin(q2) * a1 * a2 * cos(q2) - 0.3e1 * a1 ^ 2) * q2_p ^ 2 + ((a1 ^ 3 - 0.3e1 * a1 * a2 ^ 2) * cos(q2) ^ 4 + (-0.3e1 * a1 ^ 2 * a2 + a2 ^ 3) * sin(q2) * cos(q2) ^ 3 + (-0.3e1 / 0.2e1 * a1 ^ 3 + 0.5e1 / 0.2e1 * a1 * a2 ^ 2) * cos(q2) ^ 2 + 0.2e1 * cos(q2) * sin(q2) * a1 ^ 2 * a2 + a1 ^ 3 / 0.2e1) * cos(q2)) * cos(q2) * b2 * q1_pp / 0.6e1 - cos(q2) ^ 4 * b1 ^ 2 * b2 * q1_pp / (a1 * sin(q2) + a2 * cos(q2) - q2_pp) * (0.1e1 + b2 ^ 2 * q1_pp ^ 2 / b1 ^ 2 / cos(q2) ^ 2 / (a1 * sin(q2) + a2 * cos(q2) - q2_pp) ^ 2) ^ (-0.1e1 / 0.2e1) * a3 * ((a1 ^ 2 * a2 - a2 ^ 3 / 0.3e1) * cos(q2) ^ 3 + sin(q2) * a1 * (a1 ^ 2 - 0.3e1 * a2 ^ 2) * cos(q2) ^ 2 / 0.3e1 - cos(q2) * a1 ^ 2 * a2 - sin(q2) * a1 ^ 3 / 0.3e1)) * q2_pp + b2 ^ 5 * q1_pp ^ 5 / b1 / (a1 * sin(q2) + a2 * cos(q2) - q2_pp) * (0.1e1 + b2 ^ 2 * q1_pp ^ 2 / b1 ^ 2 / cos(q2) ^ 2 / (a1 * sin(q2) + a2 * cos(q2) - q2_pp) ^ 2) ^ (-0.1e1 / 0.2e1) * a3 - 0.4e1 * (cos(q2) ^ 2 * a2 + cos(q2) * sin(q2) * a1 - a2 / 0.2e1) * b1 * b2 ^ 3 * q2_p ^ 2 * q1_pp ^ 3 - 0.2e1 * cos(q2) ^ 2 * ((a1 ^ 2 - a2 ^ 2) * cos(q2) ^ 2 - 0.2e1 * sin(q2) * a1 * a2 * cos(q2) - a1 ^ 2) * b1 * b2 ^ 3 * q1_pp ^ 3 / (a1 * sin(q2) + a2 * cos(q2) - q2_pp) * (0.1e1 + b2 ^ 2 * q1_pp ^ 2 / b1 ^ 2 / cos(q2) ^ 2 / (a1 * sin(q2) + a2 * cos(q2) - q2_pp) ^ 2) ^ (-0.1e1 / 0.2e1) * a3 - 0.12e2 * b1 ^ 3 * cos(q2) * b2 * q2_p ^ 2 * ((a1 ^ 2 * a2 - a2 ^ 3 / 0.3e1) * cos(q2) ^ 5 + sin(q2) * a1 * (a1 ^ 2 - 0.3e1 * a2 ^ 2) * cos(q2) ^ 4 / 0.3e1 + (-0.3e1 / 0.2e1 * a1 ^ 2 * a2 + a2 ^ 3 / 0.2e1) * cos(q2) ^ 3 - sin(q2) * a1 * (a1 ^ 2 - 0.3e1 * a2 ^ 2) * cos(q2) ^ 2 / 0.3e1 + 0.2e1 / 0.3e1 * cos(q2) * a1 ^ 2 * a2 + sin(q2) * a1 ^ 3 / 0.6e1) * q1_pp + cos(q2) ^ 4 * b1 ^ 3 * b2 * q1_pp / (a1 * sin(q2) + a2 * cos(q2) - q2_pp) * (0.1e1 + b2 ^ 2 * q1_pp ^ 2 / b1 ^ 2 / cos(q2) ^ 2 / (a1 * sin(q2) + a2 * cos(q2) - q2_pp) ^ 2) ^ (-0.1e1 / 0.2e1) * a3 * ((a1 ^ 4 - 0.6e1 * a1 ^ 2 * a2 ^ 2 + a2 ^ 4) * cos(q2) ^ 4 + (-0.4e1 * a1 ^ 3 * a2 + 0.4e1 * a1 * a2 ^ 3) * sin(q2) * cos(q2) ^ 3 + (-0.2e1 * a1 ^ 4 + 0.6e1 * a1 ^ 2 * a2 ^ 2) * cos(q2) ^ 2 + 0.4e1 * sin(q2) * a1 ^ 3 * a2 * cos(q2) + a1 ^ 4)) / b3 / (q2_pp ^ 4 * cos(q2) ^ 4 * b1 ^ 4 - 0.4e1 * cos(q2) ^ 4 * b1 ^ 4 * (a1 * sin(q2) + a2 * cos(q2)) * q2_pp ^ 3 - 0.6e1 * b1 ^ 2 * cos(q2) ^ 2 * (-b2 ^ 2 * q1_pp ^ 2 / 0.3e1 + ((a1 ^ 2 - a2 ^ 2) * cos(q2) ^ 2 - 0.2e1 * sin(q2) * a1 * a2 * cos(q2) - a1 ^ 2) * b1 ^ 2 * cos(q2) ^ 2) * q2_pp ^ 2 + 0.12e2 * (-b2 ^ 2 * (a1 * sin(q2) + a2 * cos(q2)) * q1_pp ^ 2 / 0.3e1 + b1 ^ 2 * cos(q2) ^ 2 * ((a1 ^ 2 * a2 - a2 ^ 3 / 0.3e1) * cos(q2) ^ 3 + sin(q2) * a1 * (a1 ^ 2 - 0.3e1 * a2 ^ 2) * cos(q2) ^ 2 / 0.3e1 - cos(q2) * a1 ^ 2 * a2 - sin(q2) * a1 ^ 3 / 0.3e1)) * b1 ^ 2 * cos(q2) ^ 2 * q2_pp + b2 ^ 4 * q1_pp ^ 4 - 0.2e1 * ((a1 ^ 2 - a2 ^ 2) * cos(q2) ^ 2 - 0.2e1 * sin(q2) * a1 * a2 * cos(q2) - a1 ^ 2) * b1 ^ 2 * cos(q2) ^ 2 * b2 ^ 2 * q1_pp ^ 2 + b1 ^ 4 * cos(q2) ^ 4 * ((a1 ^ 4 - 0.6e1 * a1 ^ 2 * a2 ^ 2 + a2 ^ 4) * cos(q2) ^ 4 + (-0.4e1 * a1 ^ 3 * a2 + 0.4e1 * a1 * a2 ^ 3) * sin(q2) * cos(q2) ^ 3 + (-0.2e1 * a1 ^ 4 + 0.6e1 * a1 ^ 2 * a2 ^ 2) * cos(q2) ^ 2 + 0.4e1 * sin(q2) * a1 ^ 3 * a2 * cos(q2) + a1 ^ 4));
   
end

== matlab function Sim_Helikopter/Simulationsmodell Helikopter/F2U fb ==
  data: u input; y output
function y = fcn(u)
%#codegen

y = F2U(u(1));

== matlab function Sim_Helikopter/Simulationsmodell Helikopter/Heli/Fres ==
  data: u input; F output; parameters parameter
function F = fcn(u, parameters)
%#codegen

F = Fout(u(1),u(2),u(3),u(4),u(5),u(6),u(7),u(8),u(9),parameters);
